simulink model "Ishodnaya_model"  (R2021b)
settings: Solver=ode14x  StartTime=0.0  StopTime=2.5  FixedStep=Ts  RelTol=1e-3
values from neighbouring files (symbols this model uses):
  SYS = ss(a,b,c,d,Ts)    [vipolnenie_lr_3.m]
  Ts = 0.01    [vipolnenie_lr_3.m]
settings Model: Creator=Admin  LastModifiedBy=Admin
settings SolverCC: AlgebraicLoopSolver=TrustRegion
settings DebuggingCC: ArithmeticOperatorsInVariantConditions=warning
settings SFSimCC: CustomCodeUndefinedFunction=UseInterfaceOnly

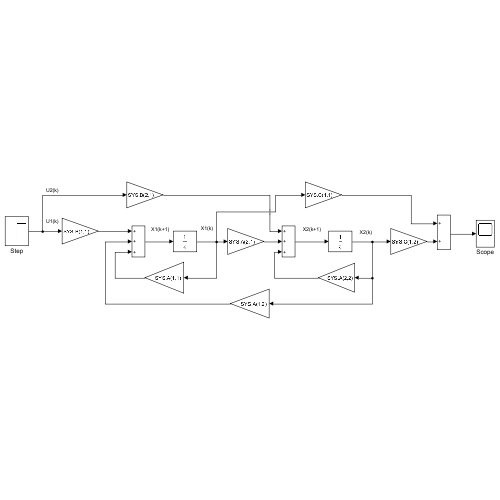
[thumbnail: Simulink's stored preview of the top-level diagram]
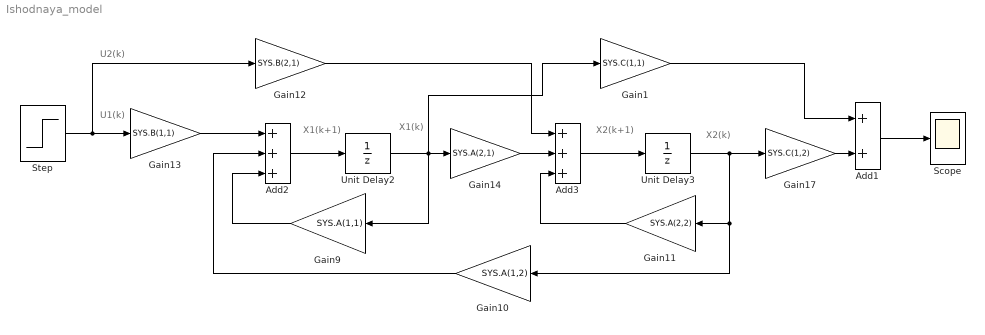
== system Ishodnaya_model ==
  note: U2(k)
  note: X1(k)
  note: X2(k)
  note: X2(k+1)
  note: X1(k+1)
  note: U1(k)
  Add1 : Sum
  Add2 : Sum  Inputs=+++
  Add3 : Sum  Inputs=+++
  Gain1 : Gain  Gain=SYS.C(1,1)
  Gain10 : Gain  Gain=SYS.A(1,2)
  Gain11 : Gain  Gain=SYS.A(2,2)
  Gain12 : Gain  Gain=SYS.B(2,1)
  Gain13 : Gain  Gain=SYS.B(1,1)
  Gain14 : Gain  Gain=SYS.A(2,1)
  Gain17 : Gain  Gain=SYS.C(1,2)
  Gain9 : Gain  Gain=SYS.A(1,1)
  Scope : Scope
  Step : Step  Time=0  SampleTime=0
  Unit Delay2 : UnitDelay  SampleTime=Ts  HasFrameUpgradeWarning=on
  Unit Delay3 : UnitDelay  SampleTime=Ts  HasFrameUpgradeWarning=on
  wires:
  Gain13/1 -> Add2/1
  Gain14/1 -> Add3/2
  Gain12/1 -> Add3/1
  Unit Delay3/1 -> Gain17/1, Gain10/1, Gain11/1
  Add2/1 -> Unit Delay2/1
  Add3/1 -> Unit Delay3/1
  Unit Delay2/1 -> Gain9/1, Gain1/1, Gain14/1
  Gain9/1 -> Add2/3
  Gain11/1 -> Add3/3
  Gain10/1 -> Add2/2
  Step/1 -> Gain12/1, Gain13/1
  Gain17/1 -> Add1/2
  Gain1/1 -> Add1/1
  Add1/1 -> Scope/1
